simulink model "pvsa"  (R2026a)
settings: Solver=VariableStepAuto
undefined symbols (not defined in the file or in its folder): w
settings Model: Creator=t0900  LastModifiedBy=t0900

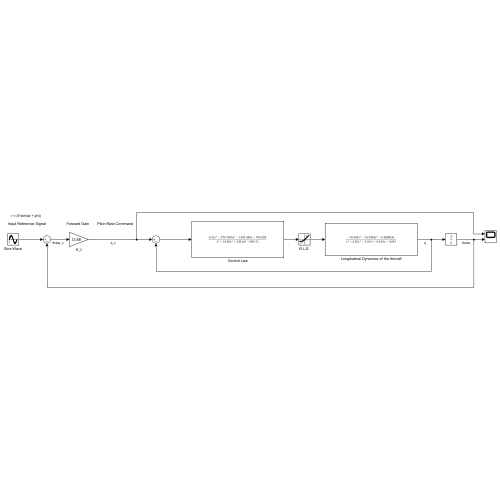
[thumbnail: Simulink's stored preview of the top-level diagram]
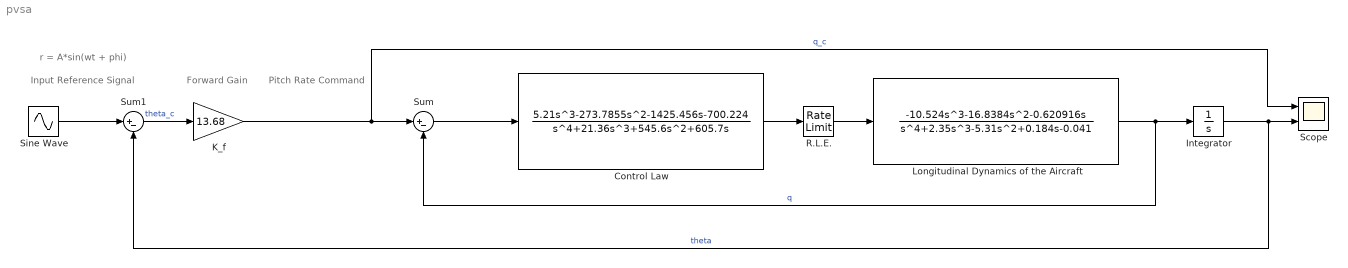
== system pvsa ==
  note: Input Reference Signal
  note: Pitch Rate Command
  note: Forward Gain
  note: r = A*sin(wt + phi)
  Control Law : TransferFcn  Numerator=[5.21, -273.7855, -1425.456, -700.224]  Denominator=[1, 21.36, 545.6, 605.7, 0]
  Integrator : Integrator
  K_f : Gain  Gain=13.68
  Longitudinal Dynamics of the Aircraft : TransferFcn  Numerator=[-10.524, -16.8384, -0.620916, 0]  Denominator=[1, 2.35, -5.31, 0.184, -0.041]
  R.L.E. : RateLimiter  RisingSlewLimit=0.707  FallingSlewLimit=-0.707  SampleTimeMode=inherited  InitialCondition=1
  Scope : Scope  NumInputPorts=2
  Sine Wave : Sin  Frequency=w  SampleTime=0
  Sum : Sum  Inputs=|+-
  Sum1 : Sum  Inputs=|+-
  wires:
  Control Law/1 -> R.L.E./1
  R.L.E./1 -> Longitudinal Dynamics of the Aircraft/1
  Sum/1 -> Control Law/1
  Longitudinal Dynamics of the Aircraft/1 -> Sum/2, Integrator/1  "q"
  K_f/1 -> Scope/1, Sum/1  "q_c"
  Integrator/1 -> Sum1/2, Scope/2  "theta"
  Sum1/1 -> K_f/1  "theta_c"
  Sine Wave/1 -> Sum1/1
